simulink model "WP1_sym"  (R2023b)
settings: Solver=VariableStepAuto  StartTime=0.0  StopTime=10.0  RelTol=1e-3
values from neighbouring files (symbols this model uses):
  K = [-1651800 2200]    [WP1.m]
undefined symbols (not defined in the file or in its folder): Kr
settings Model: Creator=kiraa  LastModifiedBy=kiraa

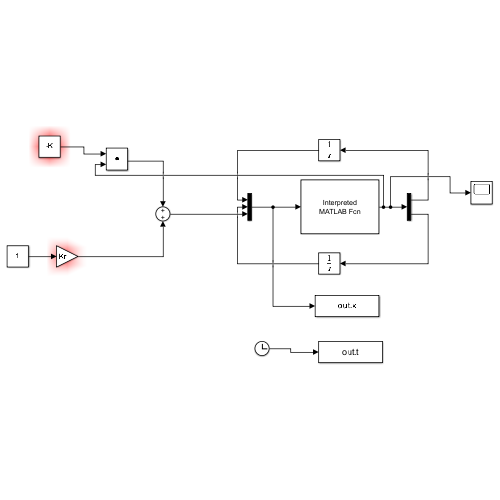
[thumbnail: Simulink's stored preview of the top-level diagram]
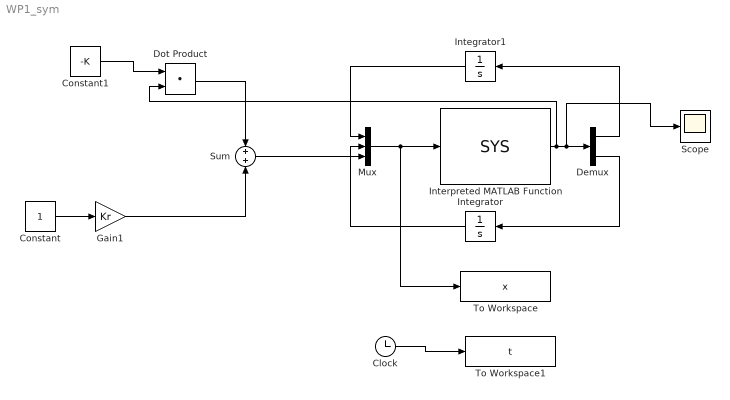
== system WP1_sym ==
  Clock : Clock
  Constant : Constant
  Constant1 : Constant  Value=-K
  Demux : Demux  Outputs=2
  Dot Product : DotProduct  OutDataTypeStr=Inherit: Inherit via internal rule
  Gain1 : Gain  Gain=Kr
  Integrator : Integrator
  Integrator1 : Integrator
  Interpreted MATLAB Function : MATLABFcn  MATLABFcn=SYS  OutputDimensions=2
  Mux : Mux  Inputs=3
  Scope : Scope
  Sum : Sum  Inputs=+|+
  To Workspace : ToWorkspace  VariableName=x  SampleTime=-1
  To Workspace1 : ToWorkspace  VariableName=t  SaveFormat=Timeseries  SampleTime=-1
  wires:
  Integrator1/1 -> Mux/1
  Clock/1 -> To Workspace1/1
  Demux/2 -> Integrator/1
  Integrator/1 -> Mux/2
  Mux/1 -> To Workspace/1, Interpreted MATLAB Function/1
  Interpreted MATLAB Function/1 -> Dot Product/2, Scope/1, Demux/1
  Demux/1 -> Integrator1/1
  Constant/1 -> Gain1/1
  Constant1/1 -> Dot Product/1
  Gain1/1 -> Sum/2
  Dot Product/1 -> Sum/1
  Sum/1 -> Mux/3
